simulink model "openloopcontrol"  (R2020a)
settings: Solver=VariableStepAuto  StartTime=0.0  StopTime=1  MaxStep=0.0001  RelTol=1e-3
libraries: powerlib x24, ECEN315_Library x13
settings Model: Creator=burmesdani  LastModifiedBy=Daniel
settings DataIOCC: ReturnWorkspaceOutputs=off
settings DebuggingCC: ArithmeticOperatorsInVariantConditions=warning
settings SFSimCC: SimUseLocalCustomCode=off  CustomCodeUndefinedFunction=UseInterfaceOnly
settings RTWCC: RTWUseLocalCustomCode=off

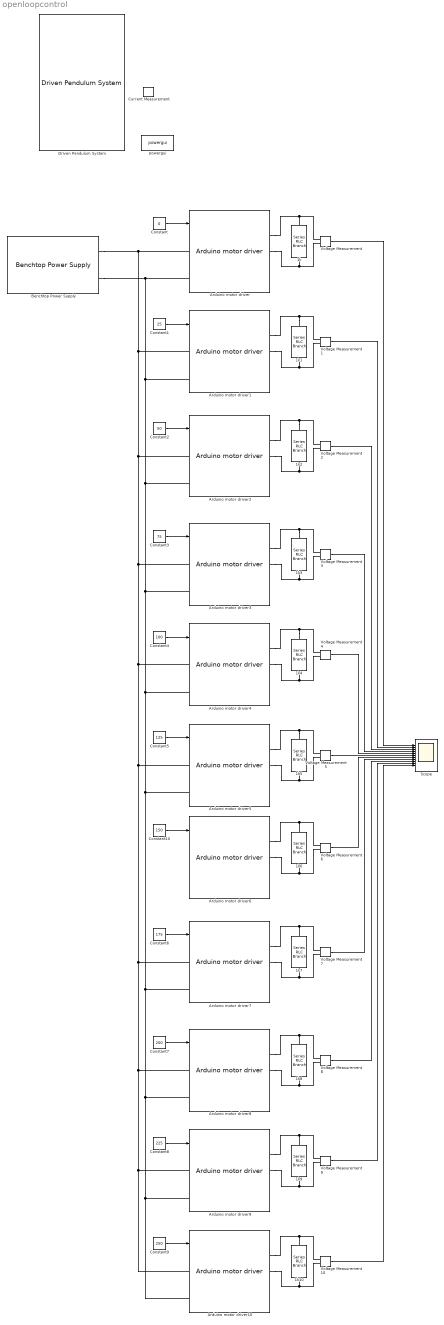
== system openloopcontrol ==
  1k{,1..10} (11 alike) : powerlib/Elements/Series RLC Branch  LConnTagsString=__new0  RConnTagsString=__new0  BranchType=R  Resistance=1000  Inductance=1e-3  SetiL0=off  InitialCurrent=0  Capacitance=1e-6  Setx0=off  InitialVoltage=0  Measurements=None
  Arduino motor driver{,1..10} (11 alike) : ECEN315_Library/Arduino motor driver  E=off
  Benchtop Power Supply : ECEN315_Library/Benchtop Power Supply  V=5
  Constant : Constant  Value=0
  Constant1 : Constant  Value=25
  Constant10 : Constant  Value=150
  Constant2 : Constant  Value=50
  Constant3 : Constant  Value=75
  Constant4 : Constant  Value=100
  Constant5 : Constant  Value=125
  Constant6 : Constant  Value=175
  Constant7 : Constant  Value=200
  Constant8 : Constant  Value=225
  Constant9 : Constant  Value=250
  Current Measurement : powerlib/Measurements/Current Measurement  PhasorSimulation=off  OutputType=Complex  PSBequivalent=0
  Driven Pendulum System : ECEN315_Library/Driven Pendulum System  SystemSampleTime=-1  Latency=0  AutoFrameSizeCalculation=off
  Scope : Scope  NumInputPorts=11
  Voltage Measurement{,1..10} (11 alike) : powerlib/Measurements/Voltage Measurement  PhasorSimulation=off  OutputType=Complex  PSBequivalent=0
  powergui : powerlib/powergui  Priority=1  SimulationMode=Continuous  SampleTime=50e-6  frequency=60  Iterations=50  frequencyindice=0  Pbase=100e6  ErrMax=1e-4  UnitsV=kV  UnitsW=MW  buscounter=0  FunctionMessages=off  echomessages=off  EnableUseOfTLC=off  CurrentSourceSwitches=off  DisableSnubberDevices=off  DisableRonSwitches=off  DisableVfSwitches=off  DisplayEquations=off  AutomaticDiscreteSolvers=off  SolverType=Tustin/Backward Euler (TBE)  Interpol=off  ExternalGateDelay=off  methode=off  Ts=100  x0status=blocks  SPID=on  SwTol=0  HookPort=off  NonlinearTolerance=1e-4  nMaxIteration=100  ContinueOnMaxIteration=off  RestoreLinks=warning  ResistiveCurrentMeasurement=off  Frange=[0:2:500]  Ylog=off  Xlog=on  ShowGrid=off  save=off  variable=ZData  structure=0  ZoomFFT=off  StartTime=0.0  cycles=1  DisplayStyle=1  fundamental=60  FreqAxis=off  MaxFrequency=1000  frequencyindicesteady=1  RmsSteady=1  display=off
  wires:
  Voltage Measurement/1 -> Scope/1
  Constant/1 -> Arduino motor driver/1
  Constant1/1 -> Arduino motor driver1/1
  Constant2/1 -> Arduino motor driver2/1
  Voltage Measurement1/1 -> Scope/2
  Voltage Measurement2/1 -> Scope/3
  Constant3/1 -> Arduino motor driver3/1
  Constant4/1 -> Arduino motor driver4/1
  Constant8/1 -> Arduino motor driver9/1
  Constant9/1 -> Arduino motor driver10/1
  Constant6/1 -> Arduino motor driver7/1
  Constant7/1 -> Arduino motor driver8/1
  Constant5/1 -> Arduino motor driver5/1
  Voltage Measurement3/1 -> Scope/4
  Voltage Measurement4/1 -> Scope/5
  Voltage Measurement5/1 -> Scope/6
  Constant10/1 -> Arduino motor driver6/1
  Voltage Measurement6/1 -> Scope/7
  Voltage Measurement7/1 -> Scope/8
  Voltage Measurement8/1 -> Scope/9
  Voltage Measurement9/1 -> Scope/10
  Voltage Measurement10/1 -> Scope/11
  connections:
  Arduino motor driver10/LConn1 -- Arduino motor driver9/LConn1 -- Arduino motor driver8/LConn1 -- Arduino motor driver7/LConn1 -- Arduino motor driver5/LConn1 -- Arduino motor driver/LConn1 -- Benchtop Power Supply/RConn1 -- Arduino motor driver1/LConn1 -- Arduino motor driver2/LConn1 -- Arduino motor driver3/LConn1 -- Arduino motor driver4/LConn1
  Arduino motor driver10/LConn2 -- Arduino motor driver9/LConn2 -- Arduino motor driver8/LConn2 -- Arduino motor driver7/LConn2 -- Arduino motor driver5/LConn2 -- Arduino motor driver/LConn2 -- Benchtop Power Supply/RConn2 -- Arduino motor driver1/LConn2 -- Arduino motor driver2/LConn2 -- Arduino motor driver3/LConn2 -- Arduino motor driver4/LConn2
  Arduino motor driver/RConn2 -- Voltage Measurement/LConn2 -- 1k/RConn1
  Arduino motor driver/RConn1 -- Voltage Measurement/LConn1 -- 1k/LConn1
  1k1/LConn1 -- Voltage Measurement1/LConn1 -- Arduino motor driver1/RConn1
  1k1/RConn1 -- Arduino motor driver1/RConn2 -- Voltage Measurement1/LConn2
  1k2/LConn1 -- Voltage Measurement2/LConn1 -- Arduino motor driver2/RConn1
  1k2/RConn1 -- Arduino motor driver2/RConn2 -- Voltage Measurement2/LConn2
  1k3/RConn1 -- Arduino motor driver3/RConn2 -- Voltage Measurement3/LConn2
  1k3/LConn1 -- Voltage Measurement3/LConn1 -- Arduino motor driver3/RConn1
  1k4/RConn1 -- Arduino motor driver4/RConn2 -- Voltage Measurement4/LConn2
  1k4/LConn1 -- Voltage Measurement4/LConn1 -- Arduino motor driver4/RConn1
  1k5/RConn1 -- Arduino motor driver5/RConn2 -- Voltage Measurement5/LConn2
  1k5/LConn1 -- Voltage Measurement5/LConn1 -- Arduino motor driver5/RConn1
  Voltage Measurement10/LConn2 -- 1k10/RConn1 -- Arduino motor driver10/RConn2
  Voltage Measurement6/LConn2 -- 1k6/RConn1 -- Arduino motor driver6/RConn2
  Voltage Measurement9/LConn2 -- 1k9/RConn1 -- Arduino motor driver9/RConn2
  Arduino motor driver8/RConn1 -- 1k8/LConn1 -- Voltage Measurement8/LConn1
  Voltage Measurement7/LConn2 -- 1k7/RConn1 -- Arduino motor driver7/RConn2
  Voltage Measurement8/LConn2 -- 1k8/RConn1 -- Arduino motor driver8/RConn2
  Arduino motor driver9/RConn1 -- 1k9/LConn1 -- Voltage Measurement9/LConn1
  Arduino motor driver7/RConn1 -- 1k7/LConn1 -- Voltage Measurement7/LConn1
  Arduino motor driver10/RConn1 -- 1k10/LConn1 -- Voltage Measurement10/LConn1
  Arduino motor driver6/RConn1 -- 1k6/LConn1 -- Voltage Measurement6/LConn1
